simulink model "stm32f4_regulardac2_demo"  (Simulink 7.3)
settings: Solver=FixedStepDiscrete  SolverMode=SingleTasking  StartTime=0.0  StopTime=0.003  RelTol=1e-3
PreLoadFcn:
  | waijung.modelPreload; % Required for working with Waijung Blockset. Do not remove.
undefined symbols (not defined in the file): A4, A5, HSEOSC, Link, LQFP176, ST, STM32F417IG
libraries: simulink x1, stm32f4_dac_lib x1, stm32f4_device_config_lib x1
CloseFcn:
  | waijung.modelClose; % Required for working with Waijung Blockset. Do not remove.
settings Model: Creator=Krisada  LastModifiedBy=Krisada
settings OptimizationCC: OptimizeModelRefInitCode=on  LifeSpan=1
settings HardwareCC: ProdEndianess=LittleEndian  ProdHWDeviceType=ARM Compatible->Cortex - M4  TargetEndianess=LittleEndian  TargetHWDeviceType=ARM Compatible->Cortex - M4
settings RTWCC: SystemTargetFile=stm32f4.tlc  GenerateMakefile=off  TemplateMakefile=ert_default_tmf  Description=STM32F4 Target  ProcessScript=stm32f4_make_rtw_hook
settings CodeAppCC: IgnoreCustomStorageClasses=off
settings STFCustomTargetCC: ModelReferenceCompliant=off  CombineOutputUpdateFcns=on  ERTCustomFileBanners=on  SupportNonInlinedSFcns=off  SystemTargetFile=stm32f4.tlc
settings ERTTargetCC: MultiwordLength=2048  ModelReferenceCompliant=off  ParMdlRefBuildCompliant=off  CompOptLevelCompliant=off  ERTFirstTimeCompliant=off  SupportContinuousTime=on  ModelStepFunctionPrototypeControlCompliant=off  CPPClassGenCompliant=off  ExtModeMexFile=noextcomm  InlinedParameterPlacement=NonHierarchical  ERTSrcFileBannerTemplate=stm32f4_code_template.cgt  ERTHdrFileBannerTemplate=stm32f4_code_template.cgt  ERTDataSrcFileTemplate=stm32f4_code_template.cgt  ERTDataHdrFileTemplate=stm32f4_code_template.cgt  ERTCustomFileTemplate=stm32f4_file_process.tlc

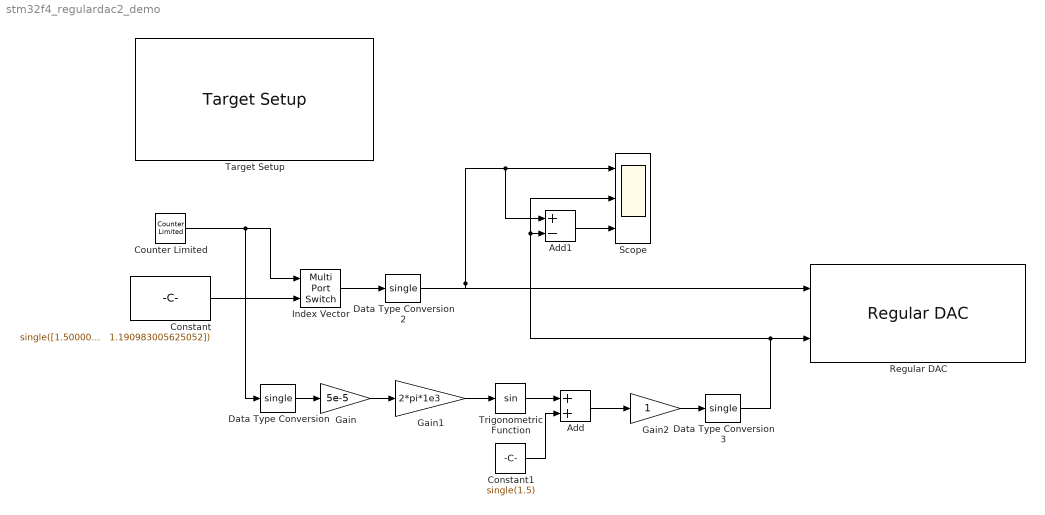
== system stm32f4_regulardac2_demo ==
  Add : Sum  OutDataType=fixdt(1, 16)  OutScaling=2^-10
  Add1 : Sum  Inputs=+-  OutDataType=fixdt(1, 16)  OutScaling=2^-10
  Constant : Constant  Value=|  OutDataType=fixdt(1, 16)  OutScaling=2^0
      | single([1.500000000000000
      |    1.809016994374948
      |    2.087785252292473
      |    2.309016994374948
      |    2.451056516295154
      |    2.500000000000000
      |    2.451056516295154
      |    2.309016994374948
      |    2.087785252292473
      |    1.809016994374948
      |    1.500000000000000
      |    1.190983005625053
      |    0.912214747707527
      |    0.690983005625053
      |    0.548943483704846
      |    0.500000000000000
      |    0.548943483704846
      |    0.690983005625052
      |    0.912214747707526
      |    1.190983005625052])
  Constant1 : Constant  Value=single(1.5)  OutDataType=fixdt(1, 16)  OutScaling=2^0
  Counter Limited : simulink/Sources/Counter Limited  SystemSampleTime=-1  uplimit=19  tsamp=5e-5
  Data Type Conversion : DataTypeConversion  OutDataTypeMode=single  OutDataType=fixdt(1, 16)  OutScaling=2^0  OutDataTypeStr=single
  Data Type Conversion2 : DataTypeConversion  OutDataTypeMode=single  OutDataType=fixdt(1, 16)  OutScaling=2^0  OutDataTypeStr=single
  Data Type Conversion3 : DataTypeConversion  OutDataTypeMode=single  OutDataType=fixdt(1, 16)  OutScaling=2^0  OutDataTypeStr=single
  Gain : Gain  Gain=5e-5  ParameterDataType=fixdt(1, 16)  ParameterScaling=2^0  OutDataType=fixdt(1, 16)  OutScaling=2^0
  Gain1 : Gain  Gain=2*pi*1e3  ParameterDataTypeMode=single  ParameterDataType=fixdt(1, 16)  ParameterScaling=2^0  ParamDataTypeStr=single  OutDataTypeMode=single  OutDataType=fixdt(1, 16)  OutScaling=2^0  OutDataTypeStr=single
  Gain2 : Gain  ParameterDataType=fixdt(1, 16)  ParameterScaling=2^0  OutDataType=fixdt(1, 16)  OutScaling=2^0
  Index Vector : MultiPortSwitch  Inputs=1  zeroidx=on  OutDataType=fixdt(1, 16)  OutScaling=2^0
  Regular DAC : stm32f4_dac_lib/Regular DAC  inputtype=Volts (single)  inputtypestr=Volts  dac1on=on  dac2on=on  advancedsettings=off  vref=3.3  dacbuffer=Enable  dacbufferstr=DAC_OutputBuffer_Enable  sampletime=-1  blockid=RegularDAC  enablecustomportlabel=off  cinputportlabel=Signal1, Signal2  coutputportlabel=0  apb=1  portpinstr=A4,A5  portstr="[\"A\"]"  pinstr="[\"GPIO_Pin_4 | GPIO_Pin_5\"]"  pinmat=[2 4 5]  chmat="[1  2]"  dacmode=DAC1_2  dacalignment=DAC_Align_12b_R  dacaddress=40007420
  Scope : Scope  NumInputPorts=3
      settings: YMin=-5~-5~-5  YMax=5~5~5
  Target Setup : stm32f4_device_config_lib/Target Setup  Priority=100  compiler=GNU ARM  previous_compiler=GNU ARM  mcu=STM32F417IG (LQFP176)  mcustr=STM32F417IG  clockconfig=HSEOSC-8MHz  system_stm32f4xx_c_path=F:\trunk\targets\stm32f4_target\stm32f4\utils\system_stm32f4xx_default\STM32F40_41xxx\hseosc8mhz  showmemoryconfiguration=on  stacksize=0x1000  heapsize=0x1000  enableautocompiledownload=on  fullchiperase=off  programmerinterface=ST-Link  editctrlstr=on  compilercontrolstr=$(patsubst %, -I%, .) -mcpu=cortex-m4 -mthumb -mthumb-interwork -mfloat-abi=hard -mfpu=fpv4-sp-d16 -ffast-math -Wall -Wextra -Ofast  assemblercontrolstr=$(patsubst %, -I%, .) -mcpu=cortex-m4 -mthumb -mthumb-interwork -mfloat-abi=hard -mfpu=fpv4-sp-d16 -ffast-math -Wall -Wextra -Ofast -Wa,-amhls=$(<:.s=.lst) -D__STACK_SIZE=$(STACK_SIZE) -D__HEAP_SIZE=$(HEAP_SIZE)  linkercontrolstr=-T$(LD_SCRIPT) -g -Wl,-Map=$(MAP),--cref,--no-warn-mismatch -mcpu=cortex-m4 -mthumb -mthumb-interwork -mfloat-abi=hard -mfpu=fpv4-sp-d16 -specs=nosys.specs  runafterdownload=on  execprofile=None  profileruart=1  profilerbaud=115200  profilertxpin=D8  profilerinitstr=1e-005,168000000,1680,115200,0  manualsetsampletime=off  sampletime=1e-005  blockid=TargetSetup  systickreloadvalue=1680  hseval=8000000  lastprofileruart=1  hclk=168000000  flashorigin=0x8000000  flashlength=1024k  ramorigin=0x20000000  ramlength=128k  useextram=off
  Trigonometric Function : Trigonometry
  wires:
  Constant/1 -> Index Vector/2
  Index Vector/1 -> Data Type Conversion2/1
  Counter Limited/1 -> Index Vector/1, Data Type Conversion/1
  Gain/1 -> Gain1/1
  Gain1/1 -> Trigonometric Function/1
  Constant1/1 -> Add/2
  Trigonometric Function/1 -> Add/1
  Add/1 -> Gain2/1
  Add1/1 -> Scope/3
  Data Type Conversion/1 -> Gain/1
  Gain2/1 -> Data Type Conversion3/1
  Data Type Conversion2/1 -> Scope/1, Add1/1, Regular DAC/1
  Data Type Conversion3/1 -> Regular DAC/2, Add1/2, Scope/2
